simulink model "T2_unstable_offset_me23b201"  (R2025a)
settings: Solver=VariableStepAuto  StartTime=0.0  StopTime=10.0  RelTol=1e-3
undefined symbols (not defined in the file or in its folder): Pm, Wcg
settings Model: Creator=abhi  LastModifiedBy=abhi

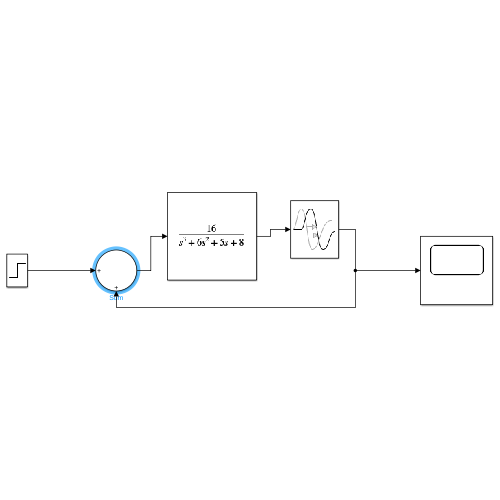
[thumbnail: Simulink's stored preview of the top-level diagram]
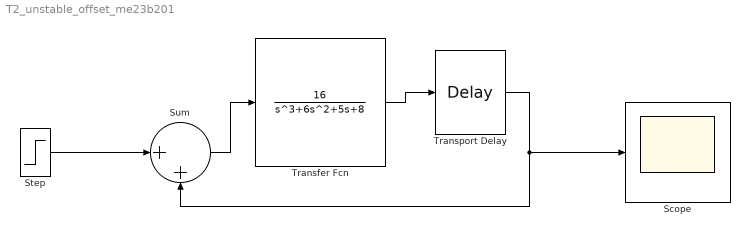
== system T2_unstable_offset_me23b201 ==
  Scope : Scope
      settings: ActiveDisplayYMinimum=-118.48057434943877  ActiveDisplayYMaximum=1066.3251691449491
  Step : Step  SampleTime=0
  Sum : Sum  Inputs=|++
  Transfer Fcn : TransferFcn  Numerator=[16]  Denominator=[1 6 5 8]
  Transport Delay : TransportDelay  DelayTime=Pm*(pi/180)/Wcg
  wires:
  Step/1 -> Sum/1
  Sum/1 -> Transfer Fcn/1
  Transfer Fcn/1 -> Transport Delay/1
  Transport Delay/1 -> Sum/2, Scope/1
